simulink model "robot_etu"  (R2022a)
settings: Solver=VariableStepAuto  StartTime=0.0  StopTime=10.0  RelTol=1e-3
values from neighbouring files (symbols this model uses):
  K = -place(A,B,[-136.4009, -2.6408, -3.5890, -5.9800])    [matrices.m]    (also in simu_robot_etu.m = [0.6700 19.9055 1.0747  1.9614])
  ue = 0    [simu_robot_etu.m]
  x0 = [0 pi/10 0 0]    [simu_robot_etu.m]
  xe = [0 0 0 0]'    [simu_robot_etu.m]
settings Model: Creator=melallem  LastModifiedBy=elgue
settings DebuggingCC: UnconnectedInputMsg=warning  UnconnectedOutputMsg=warning  UnconnectedLineMsg=warning
settings RTWCC: DLArmComputeVersion=19.05

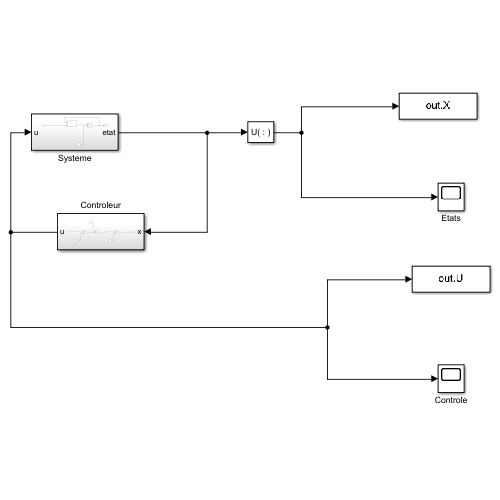
[thumbnail: Simulink's stored preview of the top-level diagram]
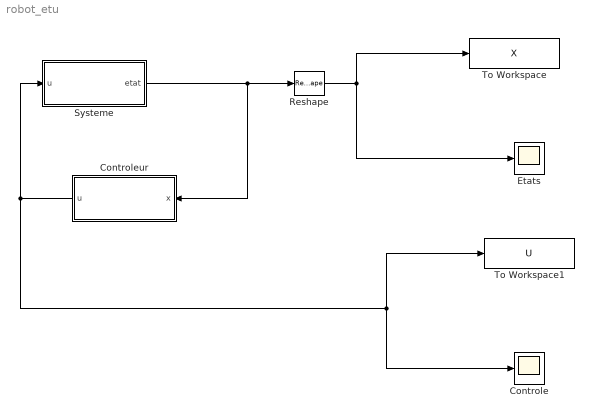
== system robot_etu ==
  Controle : Scope
  Controleur : Subsystem
  Etats : Scope
  Reshape : Reshape
  Systeme : Subsystem
  To Workspace : ToWorkspace  VariableName=X  SaveFormat=Timeseries  SampleTime=-1
  To Workspace1 : ToWorkspace  VariableName=U  SaveFormat=Timeseries  SampleTime=-1
  wires:
  Controleur/1(u) -> Controle/1, To Workspace1/1, Systeme/1(u)
  Systeme/1(etat) -> Reshape/1, Controleur/1(x)
  Reshape/1 -> Etats/1, To Workspace/1

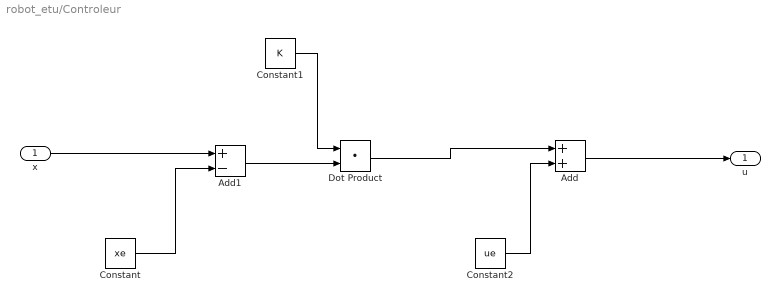
== system robot_etu/Controleur ==
  x : Inport
  Add : Sum
  Add1 : Sum  Inputs=+-
  Constant : Constant  Value=xe
  Constant1 : Constant  Value=K
  Constant2 : Constant  Value=ue
  Dot Product : DotProduct  OutDataTypeStr=Inherit: Inherit via internal rule
  u : Outport
  wires:
  x/1 -> Add1/1
  Constant/1 -> Add1/2
  Dot Product/1 -> Add/1
  Constant2/1 -> Add/2
  Add/1 -> u/1
  Constant1/1 -> Dot Product/1
  Add1/1 -> Dot Product/2

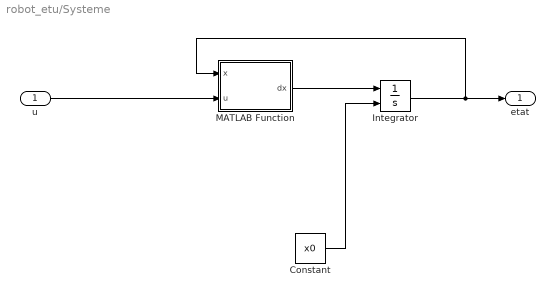
== system robot_etu/Systeme ==
  u : Inport
  Constant : Constant  Value=x0
  Integrator : Integrator  InitialConditionSource=external
  MATLAB Function : MATLAB Function  TreatAsAtomicUnit=on
  etat : Outport
  wires:
  u/1 -> MATLAB Function/2(u)
  Constant/1 -> Integrator/2
  MATLAB Function/1(dx) -> Integrator/1
  Integrator/1 -> MATLAB Function/1(x), etat/1

== matlab function robot_etu/Systeme/MATLAB Function ==
  data: x input; u input; dx output
function dx = fcn(x,u)
dx= fonction(x,u)
end
